simulink model "thermal_crap"  (Simulink 9.0)
settings: Solver=VariableStepAuto  StartTime=0.0  StopTime=10.0  RelTol=1e-3
settings Model: Creator=alibi  LastModifiedBy=alibi
settings DataIOCC: SaveFormat=Dataset
settings OptimizationCC: LifeSpan=auto
settings DebuggingCC: UnderspecifiedInitializationDetection=Simplified  MergeDetectMultiDrivingBlocksExec=error  SFUnexpectedBacktrackingDiag=error  SFNoUnconditionalDefaultTransitionDiag=error  SFExecutionAtInitializationDiag=warning
settings HardwareCC: ProdBitPerPointer=64  ProdBitPerSizeT=64  ProdBitPerPtrDiffT=64  ProdLargestAtomicFloat=Float  ProdIntDivRoundTo=Zero  ProdEndianess=LittleEndian  ProdWordSize=64  ProdHWDeviceType=Intel->x86-64 (Windows64)
settings ModelReferenceCC: PropagateSignalLabelsOutOfModel=on
settings CodeAppCC: StateflowObjectComments=off
settings GRTTargetCC: TargetLangStandard=C99 (ISO)
settings ConfigComp: CovMetricSettings=dwe  CovHtmlReporting=off  CovSaveCumulativeToWorkspaceVar=off  CovSaveSingleToWorkspaceVar=off  CovExternalEMLEnable=on

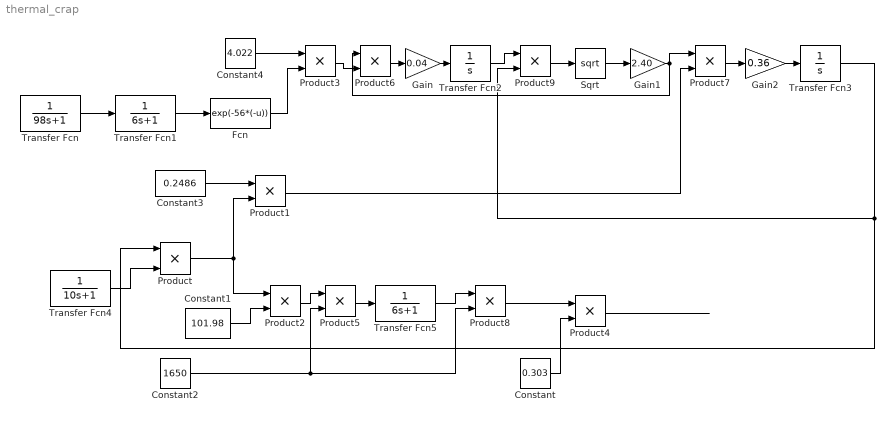
== system thermal_crap ==
  Constant : Constant  Value=0.303
  Constant1 : Constant  Value=101.98
  Constant2 : Constant  Value=1650
  Constant3 : Constant  Value=0.2486
  Constant4 : Constant  Value=4.022
  Fcn : Fcn  Expr=exp(-56*(-u))
  Gain : Gain  Gain=0.04
  Gain1 : Gain  Gain=2.40
  Gain2 : Gain  Gain=0.36
  Product : Product  Inputs=3
  Product{1..9} (9 alike) : Product
  Sqrt : Sqrt  SaturateOnIntegerOverflow=on
  Transfer Fcn : TransferFcn  Denominator=[98 1]
  Transfer Fcn1 : TransferFcn  Denominator=[6 1]
  Transfer Fcn2 : TransferFcn  Denominator=[1 0]
  Transfer Fcn3 : TransferFcn  Denominator=[1 0]
  Transfer Fcn4 : TransferFcn  Numerator=1  Denominator=[10 1]
  Transfer Fcn5 : TransferFcn  Denominator=[6 1]
  wires:
  Constant1/1 -> Product2/2
  Product/1 -> Product1/2, Product2/1
  Constant3/1 -> Product1/1
  Transfer Fcn1/1 -> Fcn/1
  Transfer Fcn/1 -> Transfer Fcn1/1
  ? -> Transfer Fcn/1
  Fcn/1 -> Product3/2
  Gain2/1 -> Transfer Fcn3/1
  Constant4/1 -> Product3/1
  Gain/1 -> Transfer Fcn2/1
  Sqrt/1 -> Gain1/1
  Gain1/1 -> Product7/1, Product6/1
  Constant/1 -> Product4/2
  Product4/1 -> ?
  Transfer Fcn4/1 -> Product/3
  ? -> Transfer Fcn4/1
  Product6/1 -> Gain/1
  Product5/1 -> Transfer Fcn5/1
  Product3/1 -> Product6/2
  Product9/1 -> Sqrt/1
  Transfer Fcn2/1 -> Product9/1
  Product8/1 -> Product4/1
  Constant2/1 -> Product5/2, Product8/2
  Transfer Fcn5/1 -> Product8/1
  Product2/1 -> Product5/1
  Transfer Fcn3/1 -> Product9/2, Product/1
  Product1/1 -> Product7/2
  Product7/1 -> Gain2/1
